simulink model "Adelanto_digital_tarea"  (R2016b)
settings: Solver=ode45  StartTime=0.0  StopTime=10  MaxStep=1e-5  RelTol=1e-3  EnableMultiTasking=on
undefined symbols (not defined in the file or in its folder): Tm
settings Model: Creator=Usuario  LastModifiedBy=Mauricio
settings DataIOCC: SaveFormat=Array  SignalLoggingSaveFormat=ModelDataLogs
settings OptimizationCC: InitFltsAndDblsToZero=on  LifeSpan=inf
settings DebuggingCC: SaveWithParameterizedLinksMsg=none  UnderspecifiedInitializationDetection=Classic  MergeDetectMultiDrivingBlocksExec=none  SignalResolutionControl=TryResolveAllWithWarning  SolverPrmCheckMsg=warning  MultiTaskDSMMsg=warning  MultiTaskCondExecSysMsg=none  FcnCallInpInsideContextMsg=warning  SFUnexpectedBacktrackingDiag=warning  SFNoUnconditionalDefaultTransitionDiag=warning  SFExecutionAtInitializationDiag=none
settings HardwareCC: ProdBitPerPointer=32  ProdBitPerSizeT=32  ProdBitPerPtrDiffT=32  ProdLargestAtomicFloat=None  ProdIntDivRoundTo=Undefined  ProdEndianess=Unspecified  ProdWordSize=32  ProdHWDeviceType=32-bit Generic
settings ModelReferenceCC: PropagateSignalLabelsOutOfModel=off
settings GRTTargetCC: TargetFcnLib=ansi_tfl_tmw.mat  TargetLangStandard=C89/C90 (ANSI)  GeneratePreprocessorConditionals=Disable all  CombineOutputUpdateFcns=off  GRTInterface=on
settings ConfigComp: CovMetricSettings=dw  CovHtmlReporting=on  CovSaveCumulativeToWorkspaceVar=on  CovSaveSingleToWorkspaceVar=on  CovExternalEMLEnable=off  CovSFcnEnable=off

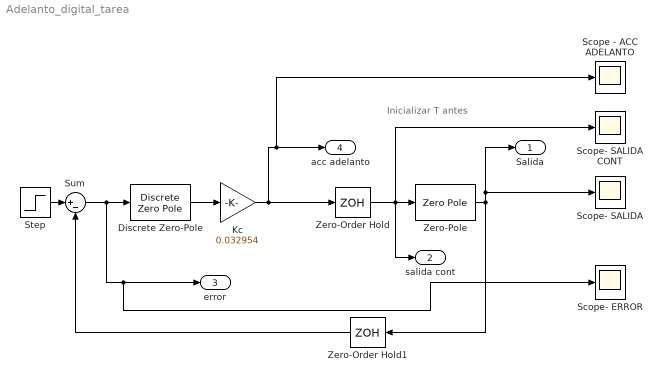
== system Adelanto_digital_tarea ==
  note: Inicializar T antes
  Discrete Zero-Pole : DiscreteZeroPole  Zeros=[0.7723]  Poles=[0.724]  Gain=1  SampleTime=Tm
  Kc : Gain  Gain=0.032954
  Scope - ACC ADELANTO : Scope
  Scope- ERROR : Scope
  Scope- SALIDA : Scope
  Scope- SALIDA CONT : Scope
  Step : Step  Time=0  SampleTime=Tm
  Sum : Sum  Inputs=|+-
  Zero-Order Hold : ZeroOrderHold  SampleTime=Tm
  Zero-Order Hold1 : ZeroOrderHold  SampleTime=Tm
  Zero-Pole : ZeroPole  Zeros=[-10]  Poles=[0 -2]  Gain=[10]
  Salida : Outport
  salida cont : Outport  Port=2
  error : Outport  Port=3
  acc adelanto : Outport  Port=4
  wires:
  Zero-Order Hold/1 -> salida cont/1, Scope- SALIDA CONT/1, Zero-Pole/1
  Step/1 -> Sum/1
  Zero-Pole/1 -> Scope- SALIDA/1, Salida/1, Zero-Order Hold1/1
  Zero-Order Hold1/1 -> Sum/2
  Sum/1 -> Discrete Zero-Pole/1, Scope- ERROR/1, error/1
  Kc/1 -> Zero-Order Hold/1, Scope - ACC ADELANTO/1, acc adelanto/1
  Discrete Zero-Pole/1 -> Kc/1
